simulink model "model_validation"  (R2020a)
settings: Solver=VariableStepAuto  StartTime=0.0  StopTime=15  RelTol=1e-3
libraries: fuzblock x4, simulink x2
settings Model: Creator=Maria  LastModifiedBy=Maria

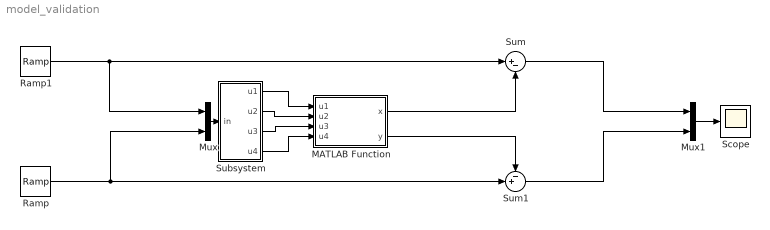
== system model_validation ==
  MATLAB Function : MATLAB Function  TreatAsAtomicUnit=on
  Mux : Mux  Inputs=2
  Mux1 : Mux  Inputs=2
  Ramp : simulink/Sources/Ramp  slope=5  start=0  InitialOutput=0  VectorParams1D=off
  Ramp1 : simulink/Sources/Ramp  slope=2  start=200  InitialOutput=0  VectorParams1D=off
  Scope : Scope
  Subsystem : Subsystem
  Sum : Sum  Inputs=|+-
  Sum1 : Sum  Inputs=-+|
  wires:
  MATLAB Function/1(x) -> Sum/2
  MATLAB Function/2(y) -> Sum1/1
  Sum/1 -> Mux1/1
  Sum1/1 -> Mux1/2
  Subsystem/1(u1) -> MATLAB Function/1(u1)
  Subsystem/2(u2) -> MATLAB Function/2(u2)
  Subsystem/3(u3) -> MATLAB Function/3(u3)
  Subsystem/4(u4) -> MATLAB Function/4(u4)
  Mux/1 -> Subsystem/1(in)
  Ramp1/1 -> Mux/1, Sum/1
  Ramp/1 -> Mux/2, Sum1/2
  Mux1/1 -> Scope/1

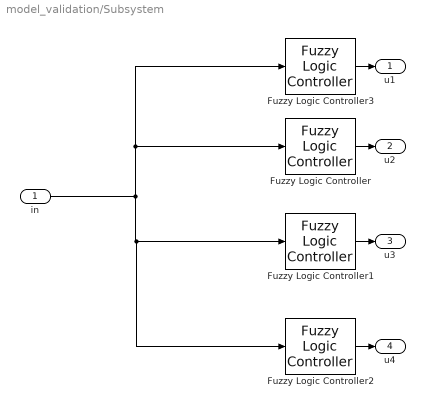
== system model_validation/Subsystem ==
  in : Inport
  Fuzzy Logic Controller : fuzblock/Fuzzy Logic  Controller  FIS=anfis2  OutputSampleNumber=101  DataType=double  FuzzifiedInputs=off  RuleFiringStrengths=off  RuleOutputs=off  AggregatedOutputs=off  SimulateUsing=Interpreted execution  OutOfRangeInputValueMessage=warning  NoRuleFiredMessage=warning  EmptyOutputFuzzySetMessage=warning
  Fuzzy Logic Controller1 : fuzblock/Fuzzy Logic  Controller  FIS=anfis3  OutputSampleNumber=101  DataType=double  FuzzifiedInputs=off  RuleFiringStrengths=off  RuleOutputs=off  AggregatedOutputs=off  SimulateUsing=Interpreted execution  OutOfRangeInputValueMessage=warning  NoRuleFiredMessage=warning  EmptyOutputFuzzySetMessage=warning
  Fuzzy Logic Controller2 : fuzblock/Fuzzy Logic  Controller  FIS=anfis4  OutputSampleNumber=101  DataType=double  FuzzifiedInputs=off  RuleFiringStrengths=off  RuleOutputs=off  AggregatedOutputs=off  SimulateUsing=Interpreted execution  OutOfRangeInputValueMessage=warning  NoRuleFiredMessage=warning  EmptyOutputFuzzySetMessage=warning
  Fuzzy Logic Controller3 : fuzblock/Fuzzy Logic  Controller  FIS=anfis1  OutputSampleNumber=101  DataType=double  FuzzifiedInputs=off  RuleFiringStrengths=off  RuleOutputs=off  AggregatedOutputs=off  SimulateUsing=Interpreted execution  OutOfRangeInputValueMessage=warning  NoRuleFiredMessage=warning  EmptyOutputFuzzySetMessage=warning
  u1 : Outport
  u2 : Outport  Port=2
  u3 : Outport  Port=3
  u4 : Outport  Port=4
  wires:
  Fuzzy Logic Controller1/1 -> u3/1
  Fuzzy Logic Controller3/1 -> u1/1
  Fuzzy Logic Controller2/1 -> u4/1
  Fuzzy Logic Controller/1 -> u2/1
  in/1 -> Fuzzy Logic Controller2/1, Fuzzy Logic Controller1/1, Fuzzy Logic Controller/1, Fuzzy Logic Controller3/1

== matlab function model_validation/MATLAB Function ==
  data: x output; u1 input; y output; u2 input; u3 input; u4 input
function [x,y] = fcn(u1,u2,u3,u4)
l1 = 105;
l2 = 55.95;
l3 = 69.07;
l4 = 14.36;

 x = l1 * cos(u1) + l2 * cos(u1 + u2) + l3 * cos(u1 + u2 + u3) + ...
     l4 * cos(u1 + u2 + u3 + u4);
 
 y = l1 * sin(u1) + l2 * sin(u1 + u2) + l3 * sin(u1 + u2 + u3) + ...
     l4 * sin(u1 + u2 + u3 + u4);

end
